simulink model "SIMULINK_watermarking"  (Simulink 7.4)
settings: Solver=ode45  StartTime=0.0  StopTime=10.0  RelTol=1e-3
undefined symbols (not defined in the file): gray, M, N, sz
libraries: vipmisc x9, viptransforms x3, vipconversions x3, vipsnks x3, vipsrcs x2
settings Model: Creator=mattwharper  LastModifiedBy=mattwharper

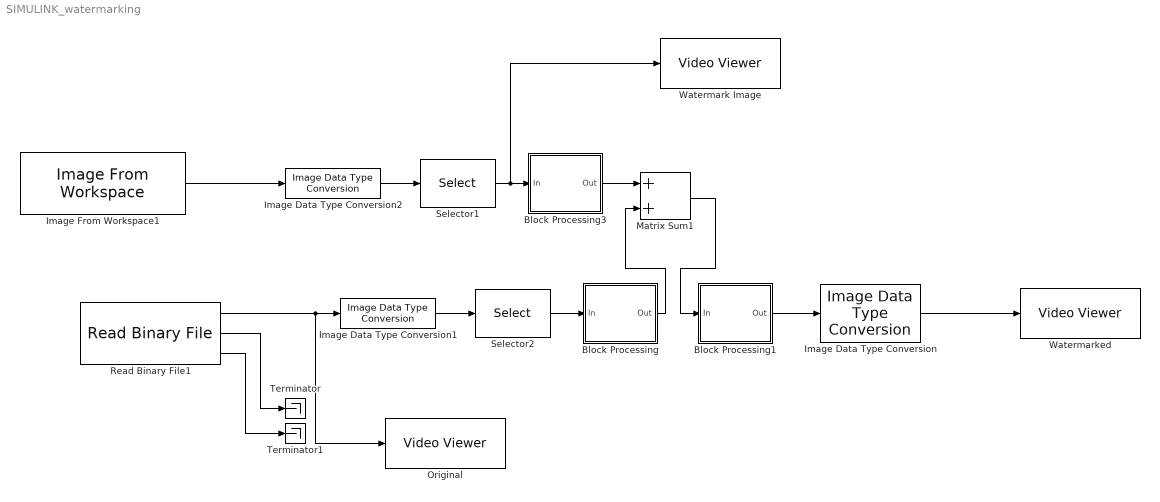
== system SIMULINK_watermarking ==
  Block Processing : Subsystem  DialogController=vipDDGCreate  DialogControllerArgs=DataTag0  TreatAsAtomicUnit=on  mask(Block Processing){NumI=1, NumO=1, Blocksize={[2 2]}, Overlapsize={[0 0]}, Traverse=Row-wise}
      mask prompts: NumI "Number of inputs:"; NumO "Number of outputs:"; Blocksize "Block size:"; Overlapsize "Overlap size:"; Traverse "Order of traversing:"
      mask help:
      | Repeats a user-specified operation on submatrices of the input matrix.
      |
      | This block extracts submatrices of a user-specified size from the input matrix. It sends each submatrix to a subsystem for processing, and then reassembles each subsystem output into the output matrix.
      |
      | Use the Block size and Overlap parameters to specify the size and overlap of each submatrix in cell array format.
      mask init:
      | errmsg = vipblkblockproc(gcbh, NumI, NumO, Blocksize, Overlapsize, Traverse);
      | error(errmsg);
      settings: CopyFcn=set_param(gcb,'LinkStatus','none');
      mask Help: eval('helpview(fullfile(docroot,''toolbox'',''vipblks'',''vipblks.map''),''vipblockprocessing'')');
      mask StyleString: edit,edit,edit,edit,popup(Row-wise|Column-wise)
      mask Display: disp('Block\n Processing');
  Block Processing1 : Subsystem  DialogController=vipDDGCreate  DialogControllerArgs=DataTag2  TreatAsAtomicUnit=on  mask(Block Processing){NumI=1, NumO=1, Blocksize={[2 2]}, Overlapsize={[0 0]}, Traverse=Row-wise}
      mask prompts: NumI "Number of inputs:"; NumO "Number of outputs:"; Blocksize "Block size:"; Overlapsize "Overlap size:"; Traverse "Order of traversing:"
      mask help:
      | Repeats a user-specified operation on submatrices of the input matrix.
      |
      | This block extracts submatrices of a user-specified size from the input matrix. It sends each submatrix to a subsystem for processing, and then reassembles each subsystem output into the output matrix.
      |
      | Use the Block size and Overlap parameters to specify the size and overlap of each submatrix in cell array format.
      mask init:
      | errmsg = vipblkblockproc(gcbh, NumI, NumO, Blocksize, Overlapsize, Traverse);
      | error(errmsg);
      settings: CopyFcn=set_param(gcb,'LinkStatus','none');
      mask Help: eval('helpview(fullfile(docroot,''toolbox'',''vipblks'',''vipblks.map''),''vipblockprocessing'')');
      mask StyleString: edit,edit,edit,edit,popup(Row-wise|Column-wise)
      mask Display: disp('Block\n Processing');
  Block Processing3 : Subsystem  DialogController=vipDDGCreate  DialogControllerArgs=DataTag4  TreatAsAtomicUnit=on  mask(Block Processing){NumI=1, NumO=1, Blocksize={[2 2]}, Overlapsize={[0 0]}, Traverse=Row-wise}
      mask prompts: NumI "Number of inputs:"; NumO "Number of outputs:"; Blocksize "Block size:"; Overlapsize "Overlap size:"; Traverse "Order of traversing:"
      mask help:
      | Repeats a user-specified operation on submatrices of the input matrix.
      |
      | This block extracts submatrices of a user-specified size from the input matrix. It sends each submatrix to a subsystem for processing, and then reassembles each subsystem output into the output matrix.
      |
      | Use the Block size and Overlap parameters to specify the size and overlap of each submatrix in cell array format.
      mask init:
      | errmsg = vipblkblockproc(gcbh, NumI, NumO, Blocksize, Overlapsize, Traverse);
      | error(errmsg);
      settings: CopyFcn=set_param(gcb,'LinkStatus','none');
      mask Help: eval('helpview(fullfile(docroot,''toolbox'',''vipblks'',''vipblks.map''),''vipblockprocessing'')');
      mask StyleString: edit,edit,edit,edit,popup(Row-wise|Column-wise)
      mask Display: disp('Block\n Processing');
  Image Data Type Conversion : vipconversions/Image Data Type Conversion  outDT=uint8  isSigned=on  wordLen=16  numFracBits=0
  Image Data Type Conversion1 : vipconversions/Image Data Type Conversion  outDT=single  isSigned=on  wordLen=16  numFracBits=0
  Image Data Type Conversion2 : vipconversions/Image Data Type Conversion  outDT=single  isSigned=on  wordLen=16  numFracBits=0
  Image From Workspace1 : vipsrcs/Image From Workspace  Tag=vipblks_nd  SystemSampleTime=-1  ImageValue=o  Ts=inf  imagePorts=One multidimensional signal  ImageDataType=Inherit from 'Value'  Signed=on  WordLength=16  sdImageDataType=sfix(16)  FractionLengthMode=User-defined  FractionLength=15  OutPortLabels=R|G|B
  Matrix Sum1 : Sum  OutDataType=sfix(16)  OutScaling=2^-10
  Original : vipsnks/Video Viewer  DialogControllerArgs=DataTag7  inputType=Obsolete7b  imagePorts=One multidimensional signal  useColorMap=off  colormapValue=gray(256)  specRange=off  minInputVal=0  maxInputVal=255  FigPos=[425 592 257 240]  AxisZoom=on  trueSizedOnce=off  OpenAtMdlStart=on
  Read Binary File1 : vipsrcs/Read Binary File  DialogController=vipDDGCreate  DialogControllerArgs=DataTag8  FileName=vipmen.bin  loopOrNot=on  numLoops=1  VideoFormat=Four character codes  FOURCC=I420  BitStreamFormat=Planar  NumOutputs=3  ComponentOrder=[1 2 3]  Interlaced=off  LineOrdering=Top line first  Ts=1/30  Component1=Y'  Component2=Cb  Component3=Cr  Component4=Alpha  Bits1=8  Bits2=8  Bits3=8  Bits4=8  Rows1=120  Rows2=60  Rows3=60  Rows4=288  Cols1=160  Cols2=80  Cols3=80  Cols4=352  YRows=120  YCols=160  SignedOutput=off  FileEndian=Little endian  OutputEOF=off
  Selector1 : Selector  NumberOfDimensions=2  IndexMode=Zero-based  InputPortWidth=3  IndexOptions=Starting index (dialog),Starting index (dialog)  Indices=0,0  OutputSizes=112,160
  Selector2 : Selector  NumberOfDimensions=2  IndexMode=Zero-based  InputPortWidth=3  IndexOptions=Starting index (dialog),Starting index (dialog)  Indices=0,0  OutputSizes=112,160
  Terminator : Terminator
  Terminator1 : Terminator
  Watermark Image : vipsnks/Video Viewer  DialogControllerArgs=DataTag10  inputType=Obsolete7b  imagePorts=One multidimensional signal  useColorMap=off  colormapValue=gray(256)  specRange=off  minInputVal=0  maxInputVal=255  FigPos=[84 340 312 263]  AxisZoom=on  trueSizedOnce=off  OpenAtMdlStart=on
  Watermarked : vipsnks/Video Viewer  DialogControllerArgs=DataTag12  inputType=Obsolete7b  imagePorts=One multidimensional signal  useColorMap=off  colormapValue=gray(256)  specRange=off  minInputVal=0  maxInputVal=255  FigPos=[604 524 325 297]  AxisZoom=on  trueSizedOnce=off  OpenAtMdlStart=on
  wires:
  Block Processing1/1(Out) -> Image Data Type Conversion/1
  Image Data Type Conversion1/1 -> Selector2/1
  Read Binary File1/2 -> Terminator/1
  Read Binary File1/3 -> Terminator1/1
  Selector2/1 -> Block Processing/1(In)
  Image Data Type Conversion/1 -> Watermarked/1
  Read Binary File1/1 -> Image Data Type Conversion1/1, Original/1
  Block Processing/1(Out) -> Matrix Sum1/2
  Matrix Sum1/1 -> Block Processing1/1(In)
  Block Processing3/1(Out) -> Matrix Sum1/1
  Selector1/1 -> Block Processing3/1(In), Watermark Image/1
  Image Data Type Conversion2/1 -> Selector1/1
  Image From Workspace1/1 -> Image Data Type Conversion2/1

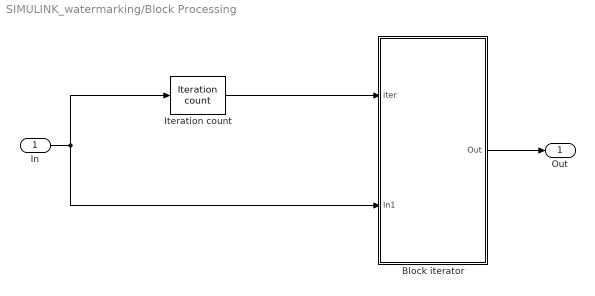
== system SIMULINK_watermarking/Block Processing ==
  In : Inport  OutDataType=sfix(16)  OutScaling=2^0
  Block iterator : Subsystem
      settings: CopyFcn=set_param(gcb,'ReferenceBlock','');
  Iteration count : vipmisc/Iteration count  blksize=Blocksize{1}  ovlpsize=Overlapsize{1}
  Out : Outport  OutDataType=sfix(16)  OutScaling=2^0
  wires:
  Iteration count/1 -> Block iterator/1(iter)
  In/1 -> Iteration count/1, Block iterator/2(In1)
  Block iterator/1(Out) -> Out/1

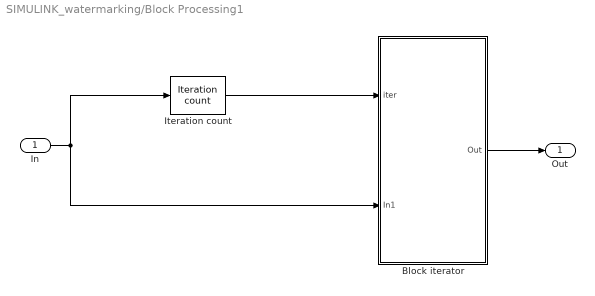
== system SIMULINK_watermarking/Block Processing1 ==
  In : Inport  OutDataType=sfix(16)  OutScaling=2^0
  Block iterator : Subsystem
      settings: CopyFcn=set_param(gcb,'ReferenceBlock','');
  Iteration count : vipmisc/Iteration count  blksize=Blocksize{1}  ovlpsize=Overlapsize{1}
  Out : Outport  OutDataType=sfix(16)  OutScaling=2^0
  wires:
  Iteration count/1 -> Block iterator/1(iter)
  In/1 -> Iteration count/1, Block iterator/2(In1)
  Block iterator/1(Out) -> Out/1

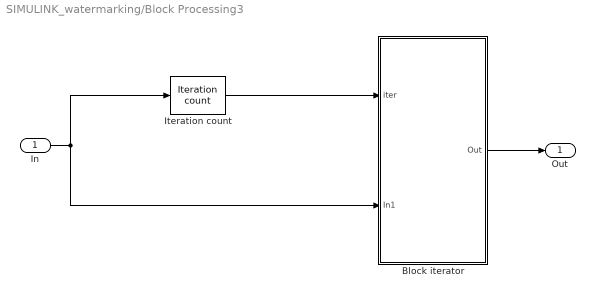
== system SIMULINK_watermarking/Block Processing3 ==
  In : Inport  OutDataType=sfix(16)  OutScaling=2^0
  Block iterator : Subsystem
      settings: CopyFcn=set_param(gcb,'ReferenceBlock','');
  Iteration count : vipmisc/Iteration count  blksize=Blocksize{1}  ovlpsize=Overlapsize{1}
  Out : Outport  OutDataType=sfix(16)  OutScaling=2^0
  wires:
  Iteration count/1 -> Block iterator/1(iter)
  In/1 -> Iteration count/1, Block iterator/2(In1)
  Block iterator/1(Out) -> Out/1

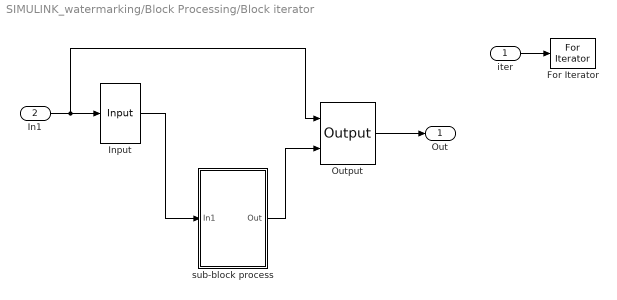
== system SIMULINK_watermarking/Block Processing/Block iterator ==
  iter : Inport  OutDataType=sfix(16)  OutScaling=2^0
  In1 : Inport  Port=2  OutDataType=sfix(16)  OutScaling=2^0
  For Iterator : ForIterator  IterationSource=external  IterationLimit=(sz(1)/M)*(sz(2)/N)  ShowIterationPort=off  IndexMode=Zero-based  IterationVariableDataType=double
  Input : vipmisc/Input  SystemSampleTime=-1  Blocksize=Blocksize{1}  Overlapsize=Overlapsize{1}  tverse=Row-wise
  Output : vipmisc/Output  SystemSampleTime=-1  Blocksize=Blocksize{1}  Overlapsize=Overlapsize{1}  tverse=Row-wise
  sub-block process : Subsystem
  Out : Outport  OutDataType=sfix(16)  OutScaling=2^0
  wires:
  iter/1 -> For Iterator/1
  In1/1 -> Output/1, Input/1
  Output/1 -> Out/1
  sub-block process/1(Out) -> Output/2
  Input/1 -> sub-block process/1(In1)

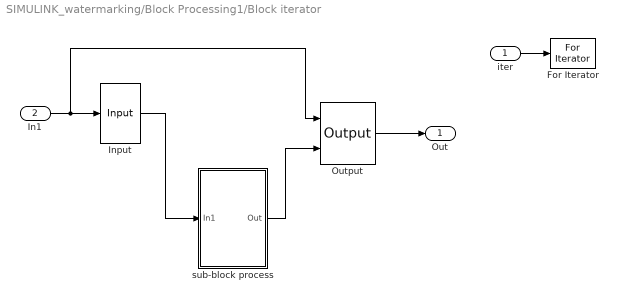
== system SIMULINK_watermarking/Block Processing1/Block iterator ==
  iter : Inport  OutDataType=sfix(16)  OutScaling=2^0
  In1 : Inport  Port=2  OutDataType=sfix(16)  OutScaling=2^0
  For Iterator : ForIterator  IterationSource=external  IterationLimit=(sz(1)/M)*(sz(2)/N)  ShowIterationPort=off  IndexMode=Zero-based  IterationVariableDataType=double
  Input : vipmisc/Input  SystemSampleTime=-1  Blocksize=Blocksize{1}  Overlapsize=Overlapsize{1}  tverse=Row-wise
  Output : vipmisc/Output  SystemSampleTime=-1  Blocksize=Blocksize{1}  Overlapsize=Overlapsize{1}  tverse=Row-wise
  sub-block process : Subsystem
  Out : Outport  OutDataType=sfix(16)  OutScaling=2^0
  wires:
  iter/1 -> For Iterator/1
  In1/1 -> Output/1, Input/1
  Output/1 -> Out/1
  sub-block process/1(Out) -> Output/2
  Input/1 -> sub-block process/1(In1)

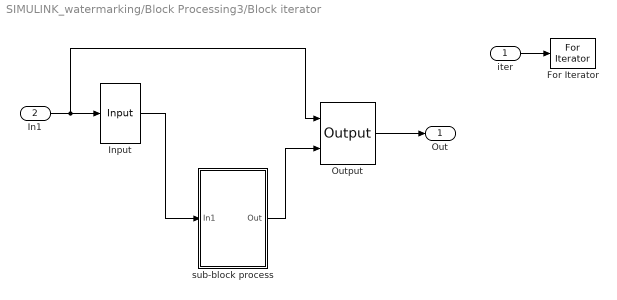
== system SIMULINK_watermarking/Block Processing3/Block iterator ==
  iter : Inport  OutDataType=sfix(16)  OutScaling=2^0
  In1 : Inport  Port=2  OutDataType=sfix(16)  OutScaling=2^0
  For Iterator : ForIterator  IterationSource=external  IterationLimit=(sz(1)/M)*(sz(2)/N)  ShowIterationPort=off  IndexMode=Zero-based  IterationVariableDataType=double
  Input : vipmisc/Input  SystemSampleTime=-1  Blocksize=Blocksize{1}  Overlapsize=Overlapsize{1}  tverse=Row-wise
  Output : vipmisc/Output  SystemSampleTime=-1  Blocksize=Blocksize{1}  Overlapsize=Overlapsize{1}  tverse=Row-wise
  sub-block process : Subsystem
  Out : Outport  OutDataType=sfix(16)  OutScaling=2^0
  wires:
  iter/1 -> For Iterator/1
  In1/1 -> Output/1, Input/1
  Output/1 -> Out/1
  sub-block process/1(Out) -> Output/2
  Input/1 -> sub-block process/1(In1)

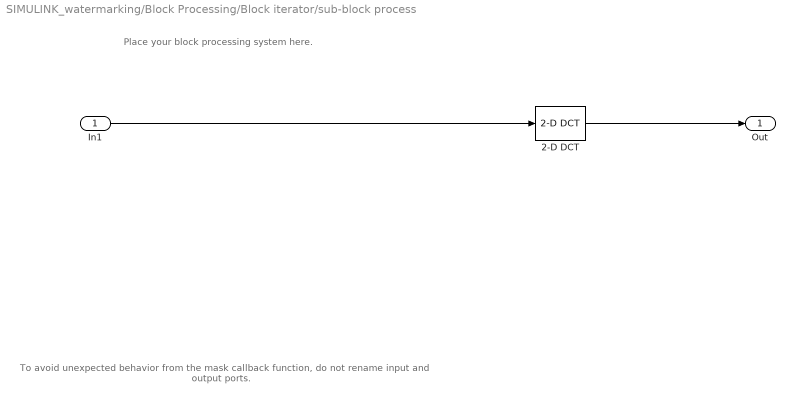
== system SIMULINK_watermarking/Block Processing/Block iterator/sub-block process ==
  note: To avoid unexpected behavior from the mask
      | callback function, do not rename input and output ports.
  note: Place your block
      | processing system here.
  In1 : Inport  OutDataType=sfix(16)  OutScaling=2^0
  2-D DCT : viptransforms/2-D DCT  DialogController=dspDDGCreate  DialogControllerArgs=DataTag1  CompMethod=Table lookup  Dimension=0  TableOpt=Speed  BitRevOrder=off  SkipNorm=off  roundingMode=Floor  overflowMode=off
  Out : Outport  OutDataType=sfix(16)  OutScaling=2^0
  wires:
  2-D DCT/1 -> Out/1
  In1/1 -> 2-D DCT/1

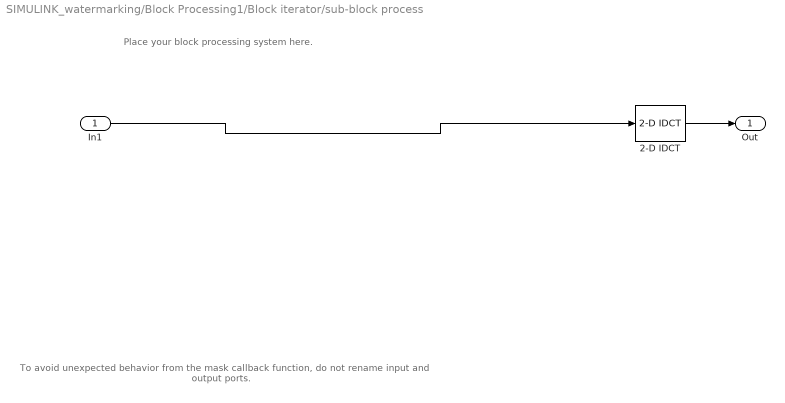
== system SIMULINK_watermarking/Block Processing1/Block iterator/sub-block process ==
  note: To avoid unexpected behavior from the mask
      | callback function, do not rename input and output ports.
  note: Place your block
      | processing system here.
  In1 : Inport  OutDataType=sfix(16)  OutScaling=2^0
  2-D IDCT : viptransforms/2-D IDCT  DialogController=dspDDGCreate  DialogControllerArgs=DataTag3  CompMethod=Table lookup  Dimension=0  TableOpt=Speed  BitRevOrder=off  SkipNorm=off  roundingMode=Floor  overflowMode=off
  Out : Outport  OutDataType=sfix(16)  OutScaling=2^0
  wires:
  2-D IDCT/1 -> Out/1
  In1/1 -> 2-D IDCT/1

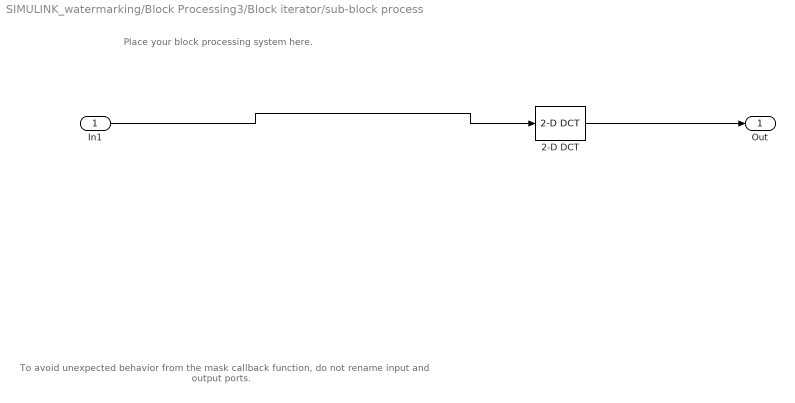
== system SIMULINK_watermarking/Block Processing3/Block iterator/sub-block process ==
  note: To avoid unexpected behavior from the mask
      | callback function, do not rename input and output ports.
  note: Place your block
      | processing system here.
  In1 : Inport  OutDataType=sfix(16)  OutScaling=2^0
  2-D DCT : viptransforms/2-D DCT  DialogController=dspDDGCreate  DialogControllerArgs=DataTag5  CompMethod=Table lookup  Dimension=0  TableOpt=Speed  BitRevOrder=off  SkipNorm=off  roundingMode=Floor  overflowMode=off
  Out : Outport  OutDataType=sfix(16)  OutScaling=2^0
  wires:
  2-D DCT/1 -> Out/1
  In1/1 -> 2-D DCT/1
